simulink model "sampleModel109"  (R2021b)
settings: Solver=VariableStepAuto  StartTime=0.0  StopTime=10.0  RelTol=1e-3
undefined symbols (not defined in the file or in its folder): DiscIntNeverNeededParam, Newton, Raphson
libraries: simulink x2, slpidlib x1
settings Model: Creator=user  LastModifiedBy=user

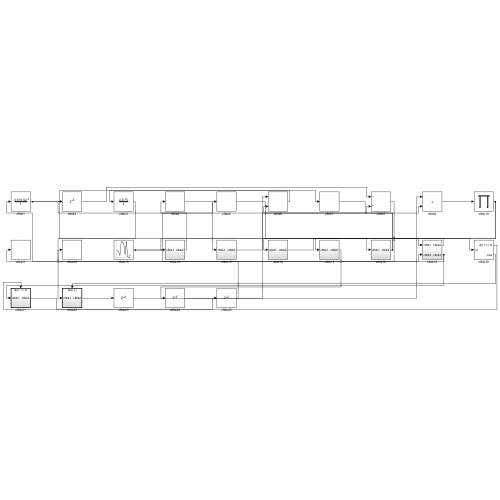
[thumbnail: Simulink's stored preview of the top-level diagram]
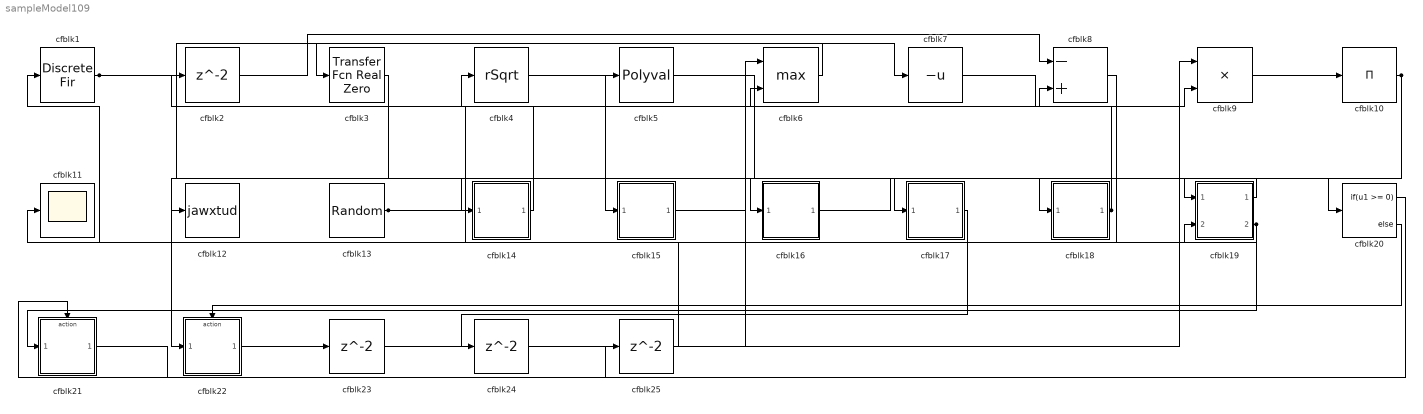
== system sampleModel109 ==
  cfblk1 : DiscreteFir  SampleTime=1
  cfblk10 : Product  Inputs=*
  cfblk11 : Scope
  cfblk12 : ToWorkspace  VariableName=jawxtud  SaveFormat=Timeseries  SampleTime=-1
  cfblk13 : RandomNumber  Mean=[-45077.482242]  Variance=[93699.322914]  Seed=[995581707.000000]  SampleTime=0.1
  cfblk14 : Subsystem
  cfblk15 : Subsystem
  cfblk16 : Subsystem
  cfblk17 : Subsystem
  cfblk18 : Subsystem
  cfblk19 : Subsystem
  cfblk{2,23..25} (4 alike) : Delay  SampleTime=1
  cfblk20 : If  IfExpression=u1 >= 0  SampleTime=1
  cfblk21 : Subsystem  TreatAsAtomicUnit=on
  cfblk22 : Subsystem  TreatAsAtomicUnit=on
  cfblk3 : simulink/Discrete/Transfer Fcn Real Zero  ZeroZ=0.75  ICPrevInput=0.0  DoSatur=off
      settings: SourceProductBaseCode=SL
  cfblk4 : Sqrt  Operator=rSqrt  AlgorithmType=Newton-Raphson  SaturateOnIntegerOverflow=on
  cfblk5 : Polyval  Coefs=[ +2.081618890e-019, -1.441693666e-014, +4.719686976e-010, -8.536869453e-006, +1.621573104e-001, -8.087801117e+001 ]
  cfblk6 : MinMax  Function=max  Inputs=2
  cfblk7 : UnaryMinus
  cfblk8 : Sum  Inputs=-+
  cfblk9 : Product  Inputs=**
  wires:
  cfblk6/1 -> cfblk3/1
  cfblk1/1 -> cfblk18/1(cfblk1), cfblk7/1
  cfblk4/1 -> cfblk15/1(cfblk1)
  cfblk8/1 -> cfblk11/1
  cfblk10/1 -> cfblk16/1(cfblk1), cfblk14/1(cfblk1)
  cfblk2/1 -> cfblk8/1
  cfblk15/1(cfblk2) -> cfblk8/2
  cfblk3/1 -> cfblk22/1(cfblk1)
  cfblk19/1(cfblk2) -> cfblk17/1(cfblk1)
  cfblk19/2(cfblk4) -> cfblk12/1, cfblk21/1(cfblk1)
  cfblk14/1(cfblk2) -> cfblk4/1
  cfblk16/1(cfblk2) -> cfblk19/1(cfblk1)
  cfblk13/1 -> cfblk19/2(cfblk3), cfblk5/1
  cfblk7/1 -> cfblk9/2
  cfblk5/1 -> cfblk20/1
  cfblk18/1(cfblk2) -> cfblk6/2, cfblk2/1
  cfblk9/1 -> cfblk10/1
  cfblk20/1 -> cfblk21/Action
  cfblk20/2 -> cfblk22/Action
  cfblk22/1(cfblk2) -> cfblk23/1
  cfblk23/1 -> cfblk6/1
  cfblk17/1(cfblk2) -> cfblk24/1
  cfblk24/1 -> cfblk9/1
  cfblk21/1(cfblk2) -> cfblk25/1
  cfblk25/1 -> cfblk1/1

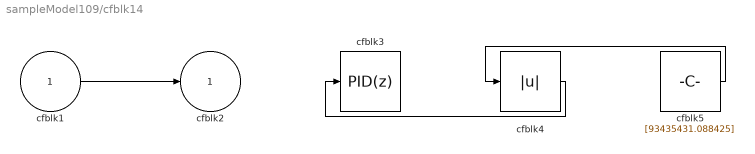
== system sampleModel109/cfblk14 ==
  cfblk1 : Inport
  cfblk3 : slpidlib/PID Controller  Controller=PID  Form=Parallel  TimeDomain=Discrete-time  UseExternalTs=off  SampleTime=1  IntegratorMethod=Forward Euler  FilterMethod=Forward Euler  ControllerParametersSource=internal  P=1  I=1  D=0  UseFilter=on  N=100  TunerSelectOption=Transfer Function Based (PID Tuner App)  InitialConditionSource=internal  InitialConditionForIntegrator=0  InitialConditionForFilter=0  DifferentiatorICPrevScaledInput=0  ExternalReset=none  TrackingMode=off  Kt=1  LimitOutput=off  SatLimitsSource=internal  UpperSaturationLimit=inf  LowerSaturationLimit=-inf  LinearizeAsGain=off  AntiWindupMode=none  Kb=1  POutMin=[]  POutMax=[]  IOutMin=[]  IOutMax=[]  DOutMin=[]  DOutMax=[]  NOutMin=[]  NOutMax=[]  SumOutMin=[]  SumOutMax=[]  SaturationOutMin=[]  SaturationOutMax=[]  PParamMin=[]  PParamMax=[]  IParamMin=[]  IParamMax=[]  DParamMin=[]  DParamMax=[]  NParamMin=[]  NParamMax=[]  KbParamMin=[]  KbParamMax=[]  KtParamMin=[]  KtParamMax=[]  KbOutMin=[]  KbOutMax=[]  KtOutMin=[]  KtOutMax=[]  IntegratorOutMin=[]  IntegratorOutMax=[]  FilterOutMin=[]  FilterOutMax=[]  SumI1OutMin=[]  SumI1OutMax=[]  SumI2OutMin=[]  SumI2OutMax=[]  SumI3OutMin=[]  SumI3OutMax=[]  SumI4OutMin=[]  SumI4OutMax=[]  SumDOutMin=[]  SumDOutMax=[]  DifferentiatorOutMin=[]  DifferentiatorOutMax=[]  FilterDiffOutCoefMin=[]  FilterDiffOutCoefMax=[]  ReciprocalOutMin=[]  ReciprocalOutMax=[]  SumDenOutMin=[]  SumDenOutMax=[]  SumNumOutMin=[]  SumNumOutMax=[]  DivideOutMin=[]  DivideOutMax=[]  UdiffTsProdOutMin=[]  UdiffTsProdOutMax=[]  NTsProdOutMin=[]  NTsProdOutMax=[]  UintegralTsProdOutMin=[]  UintegralTsProdOutMax=[]  UngainTsProdOutMin=[]  UngainTsProdOutMax=[]  IntegratorContinuousStateAttributes=''  IntegratorStateMustResolveToSignalObject=off  IntegratorRTWStateStorageClass=Auto  FilterContinuousStateAttributes=''  FilterStateMustResolveToSignalObject=off  FilterRTWStateStorageClass=Auto  ParallelPVariant=InternalParameters  IdealPVariant=Disabled  IVariant=InternalParameters  DVariant=InternalParameters  IntegratorVariant=Discrete  SatVariant=Disabled  AWVariant=Passthrough  PCopyVariant=Disabled  TRVariant=Disabled  FdbkBlocksVariant=Forward  IdealPFdbkVariant=Disabled  SatFdbkVariant=Disabled  DerivativeFilterVariant=ForwardEulerFilter  NVariant=InternalParameters  NCopyVariant=Disabled  FilterICVariant=InternalICsFilter  IntegratorICVariant=InternalICs  ExternalResetVariant=Disabled  TRSumVariant=Passthrough  SumFdbkVariant=Disabled  SumVariant=Sum_PID  TsampFilterVariant=InternalTs  TsampNgainVariant=Passthrough  TsampIntegralVariant=Passthrough  ExternalSaturationOutDataTypeStr=Inherit: Same as second input
  cfblk4 : Abs
  cfblk5 : Constant  Value=[93435431.088425]  SampleTime=1
  cfblk2 : Outport
  wires:
  cfblk5/1 -> cfblk4/1
  cfblk1/1 -> cfblk2/1
  cfblk4/1 -> cfblk3/1

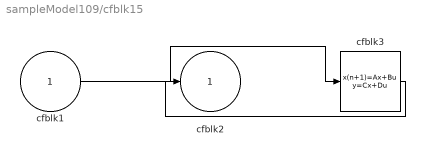
== system sampleModel109/cfblk15 ==
  cfblk1 : Inport
  cfblk3 : DiscreteStateSpace
  cfblk2 : Outport
  wires:
  cfblk1/1 -> cfblk3/1
  cfblk3/1 -> cfblk2/1

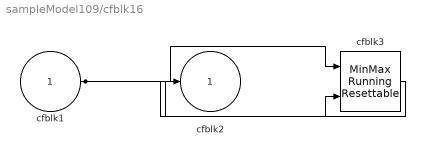
== system sampleModel109/cfblk16 ==
  cfblk1 : Inport
  cfblk3 : simulink/Math Operations/MinMax Running Resettable  Function=min  vinit=0.0
  cfblk2 : Outport
  wires:
  cfblk1/1 -> cfblk3/1, cfblk3/2
  cfblk3/1 -> cfblk2/1

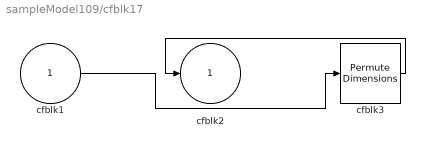
== system sampleModel109/cfblk17 ==
  cfblk1 : Inport
  cfblk3 : PermuteDimensions
  cfblk2 : Outport
  wires:
  cfblk3/1 -> cfblk2/1
  cfblk1/1 -> cfblk3/1

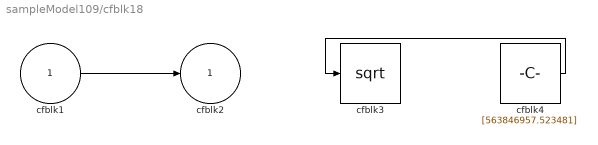
== system sampleModel109/cfblk18 ==
  cfblk1 : Inport
  cfblk3 : Sqrt  SaturateOnIntegerOverflow=on
  cfblk4 : Constant  Value=[563846957.523481]  SampleTime=1
  cfblk2 : Outport
  wires:
  cfblk1/1 -> cfblk2/1
  cfblk4/1 -> cfblk3/1

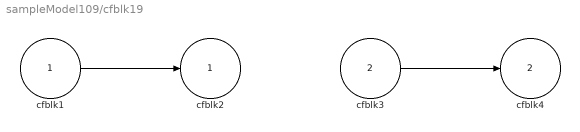
== system sampleModel109/cfblk19 ==
  cfblk1 : Inport
  cfblk3 : Inport  Port=2
  cfblk2 : Outport
  cfblk4 : Outport  Port=2
  wires:
  cfblk1/1 -> cfblk2/1
  cfblk3/1 -> cfblk4/1

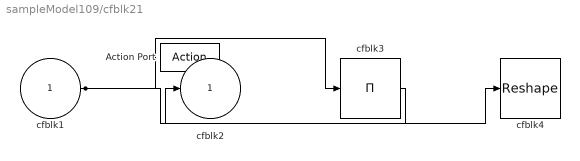
== system sampleModel109/cfblk21 ==
  cfblk1 : Inport
  Action Port : ActionPort  ActionPortLabel=if(u1 >= 0)
  cfblk3 : Product  Inputs=*
  cfblk4 : Reshape
  cfblk2 : Outport
  wires:
  cfblk3/1 -> cfblk2/1
  cfblk1/1 -> cfblk3/1, cfblk4/1

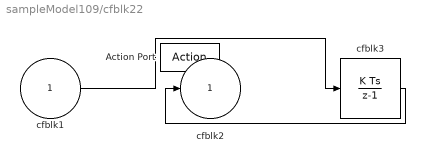
== system sampleModel109/cfblk22 ==
  cfblk1 : Inport
  Action Port : ActionPort  ActionPortLabel=else
  cfblk3 : DiscreteIntegrator  SampleTime=-1  ICPrevOutput=DiscIntNeverNeededParam  ICPrevScaledInput=DiscIntNeverNeededParam
  cfblk2 : Outport
  wires:
  cfblk3/1 -> cfblk2/1
  cfblk1/1 -> cfblk3/1
